simulink model "rail_ver01"  (R2018a)
settings: Solver=VariableStepAuto  StartTime=0.0  StopTime=inf  RelTol=1e-3
InitFcn:
  | %run('settingParams_ver04.m')
StopFcn:
  | run('AutomoveData.m')
values from neighbouring files (symbols this model uses):
  acceleration = 100    [settingParams_demo.m]
  armInitPos = [120,0,280,0,0,0,10,20]    [settingParams_demo.m]
  correct = [15, -50, 110, 35, 90, 90]    [settingParams_demo.m]
  direction = -1    [settingParams_demo.m]
  dt = 0.1    [settingParams_demo.m]
  dummyDepth = 600    [settingParams_demo.m]
  erosion = 1    [settingParams_demo.m]
  first = 0    [settingParams_demo.m]
  limit_range_ANA = [h2_1, h2_2, w2_r1, w2_r2, w2_l1, w2_l2]    [settingParams_demo.m]
  limit_range_IMG = [h1_1, h1_2, w1_r1, w1_r2, w1_l1, w1_l2]    [settingParams_demo.m]
  pitchAdd = [0,0,50,0,60,0]    [settingParams_demo.m]
  range_m = range / 1000    (= 0.9)    [settingParams_demo.m]
  range_mm = range    (= 900)    [settingParams_demo.m]
  relationOfArmCam = [530, 330, -100]    [settingParams_demo.m]
  termDistance = railDistance - robotLength - first    (= 0.8)    [settingParams_demo.m]
  translationVector = [0, 0, 0]    [settingParams_demo.m]
  value = [HMin, HMax, SMin, SMax, VMin, VMax]    [settingParams_demo.m]
  velocity = 50    [settingParams_demo.m]
undefined symbols (not defined in the file or in its folder): BodyIndexFrame, BodyTrackingID, ColorJointIndices, DepthJointIndices, gray, HandLeftConfidence, HandLeftState, HandRightConfidence, HandRightState, IsBodyTracked, JointPositions, JointTrackingState, none, serial, strel, videoinput
libraries: instrumentlib x6, simulink x4, visiontextngfix x3, visionmorphops x2, imaqlib x2, visionstatistics x1, sldrtlib x1
(part 2 of 2)

== matlab function rail_ver01/Application/Analysys Subsystem/RGBtoHAV and Binarization HSV変換と2値化 ==
  data: RGB input; BW output; value input
function BW = createMask(RGB, value)
%createMask  Threshold RGB image using auto-generated code from colorThresholder app.
%  [BW,MASKEDRGBIMAGE] = createMask(RGB) thresholds image RGB using
%  auto-generated code from the colorThresholder App. The colorspace and
%  minimum/maximum values for each channel of the colorspace were set in the
%  App and result in a binary mask BW and a composite image maskedRGBImage,
%  which shows the original RGB image values under the mask BW.

% Auto-generated by colorThresholder app on 12-Apr-2017
%------------------------------------------------------


% Convert RGB image to chosen color space
I = rgb2hsv(RGB);
%%
% H
channel1Min = value(1);
channel1Max = value(2);
% S
channel2Min = value(3);
channel2Max = value(4);
% V
channel3Min = value(5);
channel3Max = value(6);

% Create mask based on chosen histogram thresholds
sliderBW = ( (I(:,:,1) >= channel1Min) | (I(:,:,1) <= channel1Max) ) & ...
    (I(:,:,2) >= channel2Min ) & (I(:,:,2) <= channel2Max) & ...
    (I(:,:,3) >= channel3Min ) & (I(:,:,3) <= channel3Max);
%%
BW = sliderBW;

end
